simulink model "windTurbine_model"  (R2022b)
settings: Solver=VariableStepAuto  StartTime=0.0  StopTime=100  RelTol=1e-3
values from neighbouring files (symbols this model uses):
  J1 = kj * m1 * l1^2    (= 2659328)    [wind_turbine_parameters.m]
  l1 = 56    [wind_turbine_parameters.m]
  mu = 50    [wind_turbine_parameters.m]
  t_sample = 10*60    (= 600)    [wind_turbine_parameters.m]
libraries: spsWindTurbineLib x1
settings Model: Creator=luan  LastModifiedBy=luan

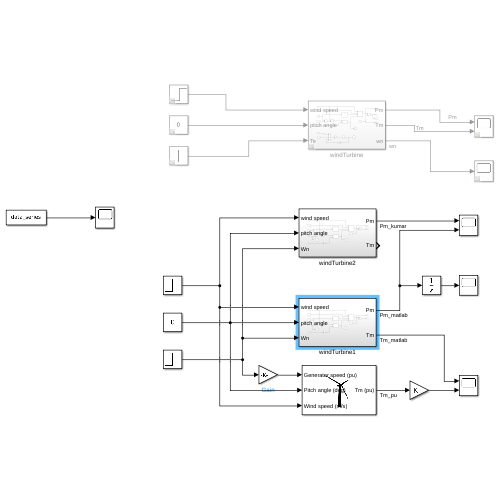
[thumbnail: Simulink's stored preview of the top-level diagram]
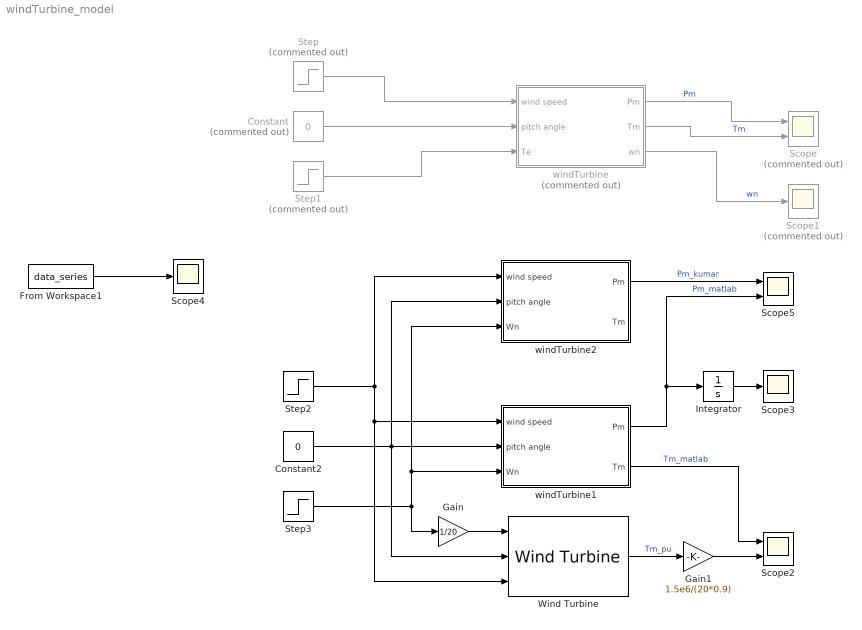
== system windTurbine_model ==
  Constant : Constant  Commented=on  Value=0
  Constant2 : Constant  Value=0
  From Workspace1 : FromWorkspace  VariableName=data_series  SampleTime=t_sample  OutputAfterFinalValue=Setting to zero
  Gain : Gain  Gain=1/20
  Gain1 : Gain  Gain=1.5e6/(20*0.9)
  Integrator : Integrator
  Scope : Scope  Commented=on  NumInputPorts=2
  Scope1 : Scope  Commented=on
  Scope2 : Scope  NumInputPorts=2
  Scope3 : Scope
  Scope4 : Scope
  Scope5 : Scope  NumInputPorts=2
  Step : Step  Commented=on  Time=0  After=18  SampleTime=0
  Step1 : Step  Commented=on  Time=5  After=50  SampleTime=0
  Step2 : Step  Time=0  After=12  SampleTime=0
  Step3 : Step  Time=0  After=15  SampleTime=0
  Wind Turbine : spsWindTurbineLib/Wind Turbine  Pnom=1.5e6  Pelec_base=1.5e6/0.9  wind_base=20  P_wind_base=0.73  speed_nom=1.2  pitch_angle=0  c1_c6="[0.51763          116          0.4            5           21     0.006795]"  cp_nom=0.48  lambda_nom=8.1
  windTurbine : Subsystem  Commented=on
  windTurbine1 : Subsystem
  windTurbine2 : Subsystem
  wires:
  Step1/1 -> windTurbine/3(Te)
  Constant/1 -> windTurbine/2(pitch angle)
  Step/1 -> windTurbine/1(wind speed)
  windTurbine/2(Tm) -> Scope/2  "Tm"
  windTurbine/1(Pm) -> Scope/1  "Pm"
  windTurbine/3(wn) -> Scope1/1  "wn"
  Step2/1 -> windTurbine1/1(wind speed), Wind Turbine/3, windTurbine2/1(wind speed)
  Constant2/1 -> Wind Turbine/2, windTurbine2/2(pitch angle), windTurbine1/2(pitch angle)
  Step3/1 -> Gain/1, windTurbine2/3(Wn), windTurbine1/3(Wn)
  Gain/1 -> Wind Turbine/1
  Wind Turbine/1 -> Gain1/1  "Tm_pu"
  windTurbine1/2(Tm) -> Scope2/1  "Tm_matlab"
  Gain1/1 -> Scope2/2
  windTurbine1/1(Pm) -> Scope5/2, Integrator/1  "Pm_matlab"
  Integrator/1 -> Scope3/1
  From Workspace1/1 -> Scope4/1
  windTurbine2/1(Pm) -> Scope5/1  "Pm_kumar"

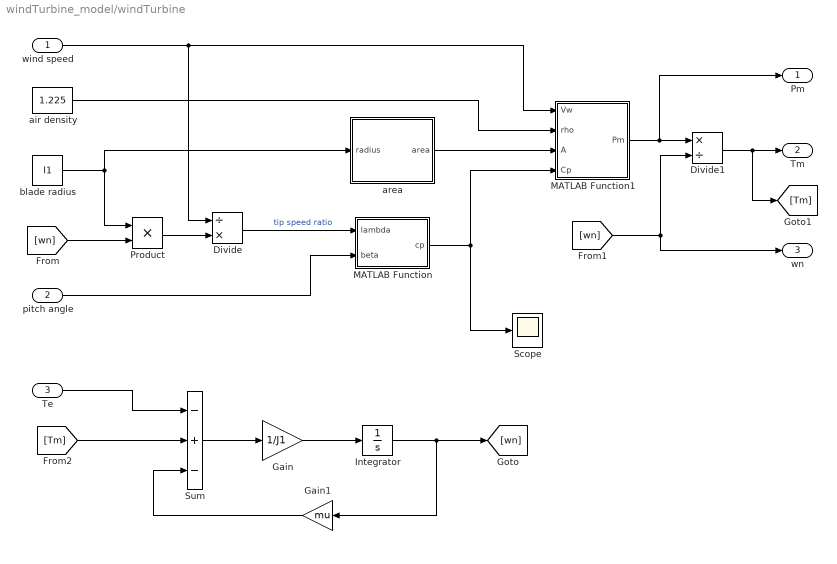
== system windTurbine_model/windTurbine ==
  wind speed : Inport
  pitch angle : Inport  Port=2
  Te : Inport  Port=3
  Divide : Product  Inputs=/*
  Divide1 : Product  Inputs=*/
  Gain : Gain  Gain=1/J1
  Gain1 : Gain  Gain=mu
  Integrator : Integrator  InitialCondition=10
  MATLAB Function : MATLAB Function  TreatAsAtomicUnit=on
  MATLAB Function1 : MATLAB Function  TreatAsAtomicUnit=on
  Product : Product
  Scope : Scope
  Sum : Sum  Inputs=-+-
  air density : Constant  Value=1.225
  area : Subsystem
  blade radius : Constant  Value=l1
  Pm : Outport
  Tm : Outport  Port=2
  wn : Outport  Port=3
  wires:
  blade radius/1 -> Product/1, area/1(radius)
  Product/1 -> Divide/2
  wind speed/1 -> MATLAB Function1/1(Vw), Divide/1
  Divide/1 -> MATLAB Function/1(lambda)  "tip speed ratio"
  pitch angle/1 -> MATLAB Function/2(beta)
  air density/1 -> MATLAB Function1/2(rho)
  area/1(area) -> MATLAB Function1/3(A)
  MATLAB Function1/1(Pm) -> Divide1/1, Pm/1
  [wn] -> wn/1, Divide1/2
  Divide1/1 -> [Tm], Tm/1
  Te/1 -> Sum/1
  [Tm] -> Sum/2
  Sum/1 -> Gain/1
  Gain/1 -> Integrator/1
  Integrator/1 -> [wn], Gain1/1
  Gain1/1 -> Sum/3
  [wn] -> Product/2
  MATLAB Function/1(cp) -> MATLAB Function1/4(Cp), Scope/1

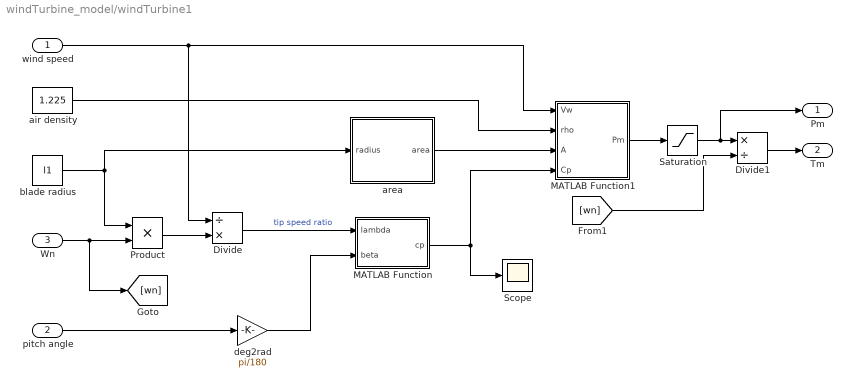
== system windTurbine_model/windTurbine1 ==
  wind speed : Inport
  pitch angle : Inport  Port=2
  Wn : Inport  Port=3
  Divide : Product  Inputs=/*
  Divide1 : Product  Inputs=*/
  MATLAB Function : MATLAB Function  TreatAsAtomicUnit=on
  MATLAB Function1 : MATLAB Function  TreatAsAtomicUnit=on
  Product : Product
  Saturation : Saturate  UpperLimit=inf  LowerLimit=0
  Scope : Scope
  air density : Constant  Value=1.225
  area : Subsystem
  blade radius : Constant  Value=l1
  deg2rad : Gain  Gain=pi/180
  Pm : Outport
  Tm : Outport  Port=2
  wires:
  MATLAB Function/1(cp) -> Scope/1, MATLAB Function1/4(Cp)
  Wn/1 -> [wn], Product/2
  Divide1/1 -> Tm/1
  [wn] -> Divide1/2
  MATLAB Function1/1(Pm) -> Saturation/1
  area/1(area) -> MATLAB Function1/3(A)
  air density/1 -> MATLAB Function1/2(rho)
  pitch angle/1 -> deg2rad/1
  Divide/1 -> MATLAB Function/1(lambda)  "tip speed ratio"
  wind speed/1 -> Divide/1, MATLAB Function1/1(Vw)
  Product/1 -> Divide/2
  blade radius/1 -> area/1(radius), Product/1
  deg2rad/1 -> MATLAB Function/2(beta)
  Saturation/1 -> Pm/1, Divide1/1

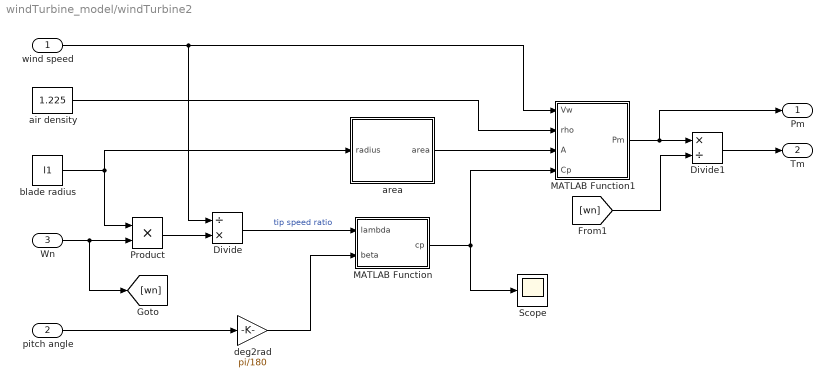
== system windTurbine_model/windTurbine2 ==
  wind speed : Inport
  pitch angle : Inport  Port=2
  Wn : Inport  Port=3
  Divide : Product  Inputs=/*
  Divide1 : Product  Inputs=*/
  MATLAB Function : MATLAB Function  TreatAsAtomicUnit=on
  MATLAB Function1 : MATLAB Function  TreatAsAtomicUnit=on
  Product : Product
  Scope : Scope
  air density : Constant  Value=1.225
  area : Subsystem
  blade radius : Constant  Value=l1
  deg2rad : Gain  Gain=pi/180
  Pm : Outport
  Tm : Outport  Port=2
  wires:
  deg2rad/1 -> MATLAB Function/2(beta)
  blade radius/1 -> Product/1, area/1(radius)
  Product/1 -> Divide/2
  wind speed/1 -> MATLAB Function1/1(Vw), Divide/1
  Divide/1 -> MATLAB Function/1(lambda)  "tip speed ratio"
  pitch angle/1 -> deg2rad/1
  air density/1 -> MATLAB Function1/2(rho)
  area/1(area) -> MATLAB Function1/3(A)
  MATLAB Function1/1(Pm) -> Divide1/1, Pm/1
  [wn] -> Divide1/2
  Divide1/1 -> Tm/1
  Wn/1 -> Product/2, [wn]
  MATLAB Function/1(cp) -> Scope/1, MATLAB Function1/4(Cp)

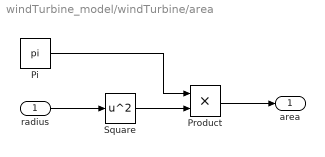
== system windTurbine_model/windTurbine/area ==
  radius : Inport
  Pi : Constant  Value=pi  OutDataTypeStr=Inherit: Inherit via back propagation
  Product : Product
  Square : Math  Operator=square
  area : Outport
  wires:
  radius/1 -> Square/1
  Square/1 -> Product/2
  Pi/1 -> Product/1
  Product/1 -> area/1

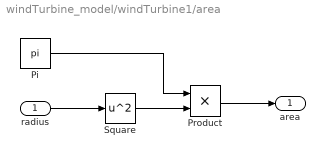
== system windTurbine_model/windTurbine1/area ==
  radius : Inport
  Pi : Constant  Value=pi  OutDataTypeStr=Inherit: Inherit via back propagation
  Product : Product
  Square : Math  Operator=square
  area : Outport
  wires:
  Product/1 -> area/1
  Pi/1 -> Product/1
  Square/1 -> Product/2
  radius/1 -> Square/1

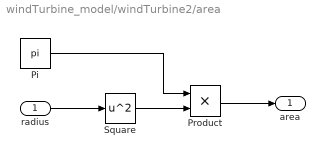
== system windTurbine_model/windTurbine2/area ==
  radius : Inport
  Pi : Constant  Value=pi  OutDataTypeStr=Inherit: Inherit via back propagation
  Product : Product
  Square : Math  Operator=square
  area : Outport
  wires:
  radius/1 -> Square/1
  Square/1 -> Product/2
  Pi/1 -> Product/1
  Product/1 -> area/1

== matlab function windTurbine_model/windTurbine/MATLAB Function1 ==
  data: Vw input; Pm output; rho input; A input; Cp input
function Pm = fcn(Vw, rho, A, Cp)

Pm = 0.5* Cp* rho* A* Vw^3;

== matlab function windTurbine_model/windTurbine/MATLAB Function ==
  data: lambda input; cp output; beta input
function cp = fcn(lambda, beta)

k = load('coefficients.mat');
lambda_i =  (1/(lambda + 0.08*beta) - 0.035/(1+beta^3))^(-1);
cp = k.k1 *(k.k2/lambda_i - k.k3*beta - k.k4*beta^(k.k5) -k.k6)*exp(-k.k7/lambda_i);

== matlab function windTurbine_model/windTurbine1/MATLAB Function ==
  data: lambda input; cp output; beta input
function cp = fcn(lambda, beta)

model = 'matlab_model';

if(strcmp(model, 'kumar_model'))
    %disp(model)
    k = load('coefficients.mat');
    lambda_i =  1/(1/(lambda + 0.08*beta) - 0.035/(1+beta^3));
    cp = k.k1 *(k.k2/lambda_i - k.k3*beta - k.k4*beta^(k.k5) -k.k6)*exp(-k.k7/lambda_i);
end
if(strcmp(model, 'matlab_model'))
    %disp(model)
    k = load('coefficients_matlab_model.mat');
    lambda_i =  1/(1/(lambda + 0.08*beta) - 0.035/(1+beta^3));
    cp = k.k1*( k.k2/lambda_i - k.k3*beta - k.k4 )*exp( -k.k5/lambda_i ) + k.k6*lambda;
end

== matlab function windTurbine_model/windTurbine1/MATLAB Function1 ==
  data: Vw input; Pm output; rho input; A input; Cp input
function Pm = fcn(Vw, rho, A, Cp)

Pm = 0.5* Cp* rho* A* Vw^3;

== matlab function windTurbine_model/windTurbine2/MATLAB Function ==
  data: lambda input; cp output; beta input
function cp = fcn(lambda, beta)

model = 'kumar_model';

if(strcmp(model, 'kumar_model'))
    %disp(model)
    k = load('coefficients.mat');
    lambda_i =  1/(1/(lambda + 0.08*beta) - 0.035/(1+beta^3));
    cp = k.k1 *(k.k2/lambda_i - k.k3*beta - k.k4*beta^(k.k5) -k.k6)*exp(-k.k7/lambda_i);
end
if(strcmp(model, 'matlab_model'))
    %disp(model)
    k = load('coefficients_matlab_model.mat');
    lambda_i =  1/(1/(lambda + 0.08*beta) - 0.035/(1+beta^3));
    cp = k.k1*( k.k2/lambda_i - k.k3*beta - k.k4 )*exp( -k.k5/lambda_i ) + k.k6*lambda;
end

== matlab function windTurbine_model/windTurbine2/MATLAB Function1 ==
  data: Vw input; Pm output; rho input; A input; Cp input
function Pm = fcn(Vw, rho, A, Cp)

Pm = 0.5* Cp* rho* A* Vw^3;
